simulink model "model1"  (R2015a)
settings: Solver=ode45  SolverMode=SingleTasking  StartTime=0.0  StopTime=10.0  RelTol=1e-3
values from neighbouring files (symbols this model uses):
  adapt = 1    [init.m]    (also in init_model.m; init_mussels.m; init_mussels_2.m; init_mussels_konfiguracija_blizu.m)
  c = [ 0   0.2   0   0   0 ... (first row only)    [init.m]    (also in init_mussels.m = zeros(n,n); init_mussels_2.m; init_mussels_konfiguracija_blizu.m = [ 0   0.2   0.7   0.8   0.9; init_mussels_konfiguracija_daleko.m = [ 0   0.2   0.7   0.8   0.9)
  K = 0.02    [init.m]    (also in init_model.m; init_mussels.m; init_mussels_2.m; init_mussels_konfiguracija_blizu.m)
  sigma_0 = [ 0    0.7   0    0    0 ... (first row only)    [init.m]    (also in init_model.m = zeros(M,M); init_mussels.m = zeros(n,n); init_mussels_2.m; init_mussels_konfiguracija_blizu.m = [ 0    0.7   0.4    0.6    0.5)
  speed = zeros(3,n)    [init_mussels.m]    (also in init_mussels_2.m; init_mussels_konfiguracija_blizu.m; init_mussels_konfiguracija_daleko.m; init_mussels_konfiguracija_srednje.m)
  zeta_0 = zeros(n,n)    [init.m]    (also in init_model.m = zeros(M,M); init_mussels.m; init_mussels_2.m; init_mussels_konfiguracija_blizu.m)
settings Model: Creator=Marta_2805  LastModifiedBy=Barbara
settings OptimizationCC: BlockReduction=off  BooleanDataType=off
settings DebuggingCC: SaveWithParameterizedLinksMsg=none  UnderspecifiedInitializationDetection=Classic  MergeDetectMultiDrivingBlocksExec=none  SignalResolutionControl=TryResolveAllWithWarning
settings HardwareCC: TargetUnknown=on

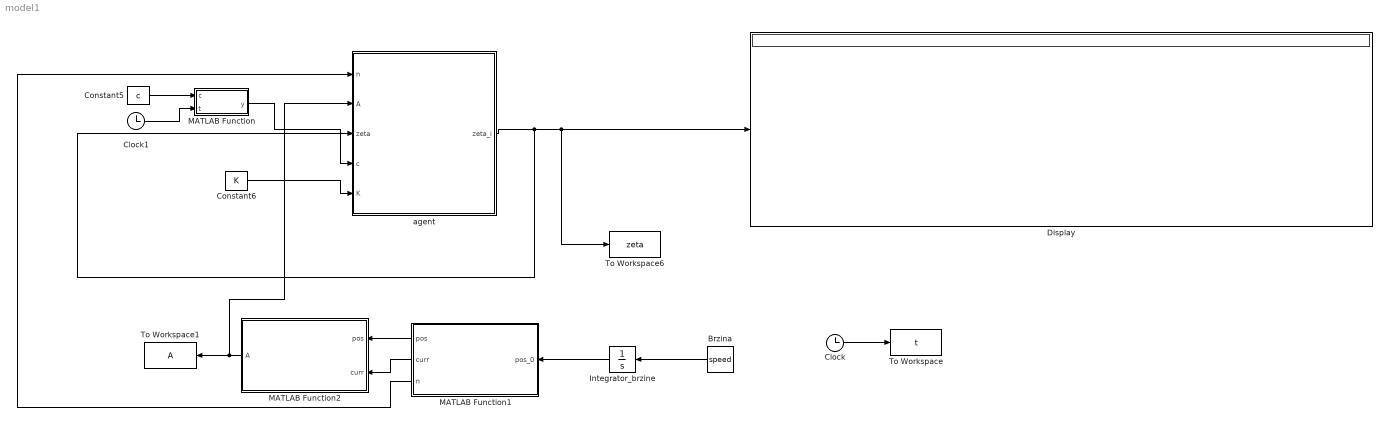
== system model1 ==
  Brzina : Constant  Value=speed  SampleTime=-1
  Clock : Clock
  Clock1 : Clock
  Constant5 : Constant  Value=c
  Constant6 : Constant  Value=K
  Display : Display
  Integrator_brzine : Integrator  InitialCondition=[0 0 0 0 0;0 0 0 0 0;0 0 0 0 0]
  MATLAB Function : MATLAB Function  TreatAsAtomicUnit=on
  MATLAB Function1 : MATLAB Function  TreatAsAtomicUnit=on
  MATLAB Function2 : MATLAB Function  TreatAsAtomicUnit=on
  To Workspace : ToWorkspace  VariableName=t  SampleTime=-1
  To Workspace1 : ToWorkspace  VariableName=A  SampleTime=-1
  To Workspace6 : ToWorkspace  VariableName=zeta  SampleTime=-1
  "agent " : Subsystem
  wires:
  Constant6/1 -> "agent "/5(K)
  MATLAB Function/1(y) -> "agent "/4(c)
  "agent "/1(zeta_i) -> "agent "/3(zeta), Display/1, To Workspace6/1
  Clock/1 -> To Workspace/1
  Constant5/1 -> MATLAB Function/1(c)
  Clock1/1 -> MATLAB Function/2(t)
  MATLAB Function1/1(pos) -> MATLAB Function2/1(pos)
  MATLAB Function1/2(curr) -> MATLAB Function2/2(curr)
  MATLAB Function2/1(A) -> To Workspace1/1, "agent "/2(A)
  MATLAB Function1/3(n) -> "agent "/1(n)
  Integrator_brzine/1 -> MATLAB Function1/1(pos_0)
  Brzina/1 -> Integrator_brzine/1

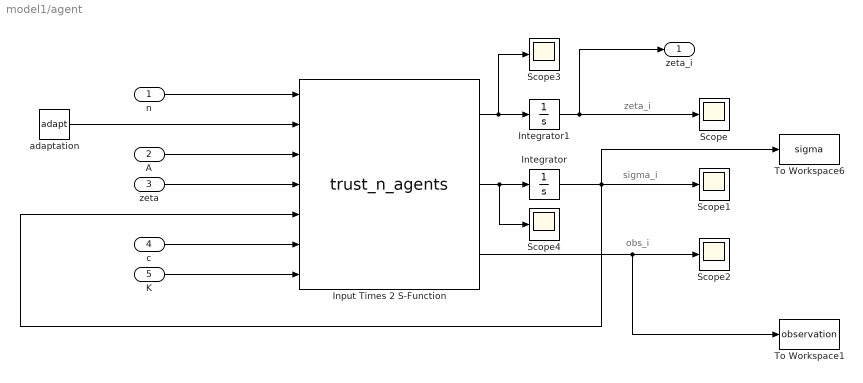
== system model1/agent  ==
  note: obs_i
  note: sigma_i
  note: zeta_i
  n : Inport
  A : Inport  Port=2
  zeta : Inport  Port=3
  c : Inport  Port=4
  K : Inport  Port=5
  Input Times 2 S-Function : S-Function  FunctionName=trust_n_agents
  Integrator : Integrator  InitialCondition=sigma_0
  Integrator1 : Integrator  InitialCondition=zeta_0
  Scope{,1..4} (5 alike) : Scope
      Scope settings: TimeRange=20  YMin=0.25  YMax=0.95
      Scope2 settings: YMin=0  YMax=0.2  SaveName=ScopeData2
      Scope3 settings: TimeRange=20  YMin=0.25  YMax=0.95  SaveName=ScopeData3
      Scope4 settings: TimeRange=20  YMin=0.25  YMax=0.95  SaveName=ScopeData4
  To Workspace1 : ToWorkspace  VariableName=observation  SampleTime=-1
  To Workspace6 : ToWorkspace  VariableName=sigma  SampleTime=-1
  adaptation : Constant  Value=adapt
  zeta_i : Outport
  wires:
  Integrator/1 -> Input Times 2 S-Function/5, To Workspace6/1, Scope1/1
  Integrator1/1 -> zeta_i/1, Scope/1
  c/1 -> Input Times 2 S-Function/6
  K/1 -> Input Times 2 S-Function/7
  Input Times 2 S-Function/2 -> Scope4/1, Integrator/1
  Input Times 2 S-Function/1 -> Scope3/1, Integrator1/1
  Input Times 2 S-Function/3 -> To Workspace1/1, Scope2/1
  n/1 -> Input Times 2 S-Function/1
  adaptation/1 -> Input Times 2 S-Function/2
  zeta/1 -> Input Times 2 S-Function/4
  A/1 -> Input Times 2 S-Function/3

== matlab function model1/MATLAB Function2 ==
  data: pos input; curr input; A output
function A  = scenario(pos, curr)
%#codegen
%radijus komunikacije
r = 0.01;

n=length(pos);
%[m,n] = size(pos);
%inicijalizacija matrice A
A=zeros(n);

for i = 1:n
    for j = 1:n
        %odredivanje udaljenosti izmedju musula - prvo x, y, pa z
        distance = sqrt((pos(1,i)-pos(1,j))^2 + (pos(2,i)-pos(2,j))^2+(pos(3,i)-pos(3,j))^2);
        
        %provjera mogu li komunicirati
        if distance < r
            
            %element ne komunicira sam sa sobom
            if i == j
                A(i,j) = 0;
            else
                A(i,j) = 1;
            end
                        
        else
            A(i,j) = 0;
        end
        
    end
       
end


end

== matlab function model1/MATLAB Function1 ==
  data: pos output; curr output; n output; pos_0 input
function [pos, curr, n] = mussels (pos_0)
%#codegen
%u inpute bi trebalo dodati koordinate, deltu i zetu?

n=5;
pos = pos_0;

X = zeros(1,n);
Y = zeros(1,n);
Z = zeros(1,n);

%mussels su blizu jedna druge
%{
X(1) = 1;
Y(1) = 1;
Z = zeros(1,n);

for i = 2 : n
    
    X(i) = X(i-1)+0.1;
    Y(i) = Y(i-1)+0.1;

end
%}
%mussels su rasprsene


X(1) = 1;
Y(1) = 1;
Z = zeros(1,n);

for i = 2 : n
    
    X(i) = X(i-1)+10;
    Y(i) = Y(i-1)+10;

end


%{
%random postavljanje koordinata
X = randperm(15,n); 
Y = randperm(15,n);
Z = zeros(1,n);
%}

%stvaranje matrice pozicije
    pos(1,:) = X;
    pos(2,:) = Y;
    pos(3,:) = Z;

%mjerenja
curr = randi(3,size(X));

end

== matlab function model1/MATLAB Function ==
  data: c input; y output; t input
function y = fcn(c, t)
%#codegen
if t > 25
    c(:,1) = c(:,1);
%    c(:,13) = c(:,13) / 5; 
%    c(:,13) = c(:,13) / 7;
%    c(:,3) = c(:,3) * 2;
end
y = c;
